simulink library "baro_block_visual"  (R2025b)
settings: Solver=VariableStepAuto  StartTime=0.0  StopTime=10.0  RelTol=1e-3
values from neighbouring files (symbols this model uses):
  Baro = evalin('base', 'Baro')    [casper_baro_step.m]    (also in test_baro_model.m)
  Sim = evalin('base', 'Sim')    [casper_baro_step.m]    (also in test_baro_model.m)
settings Model: Creator=Ashwin  LastModifiedBy=Ashwin

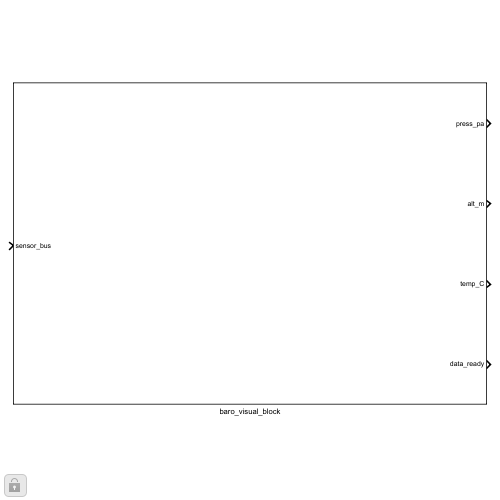
[thumbnail: Simulink's stored preview of the top-level diagram]
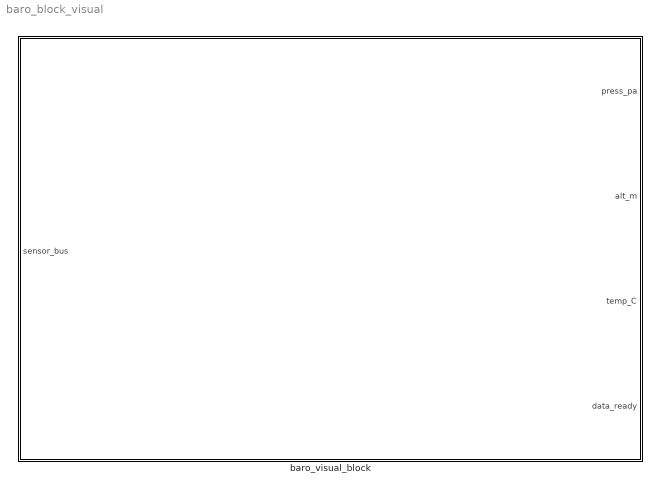
== system baro_block_visual ==
  baro_visual_block : Subsystem

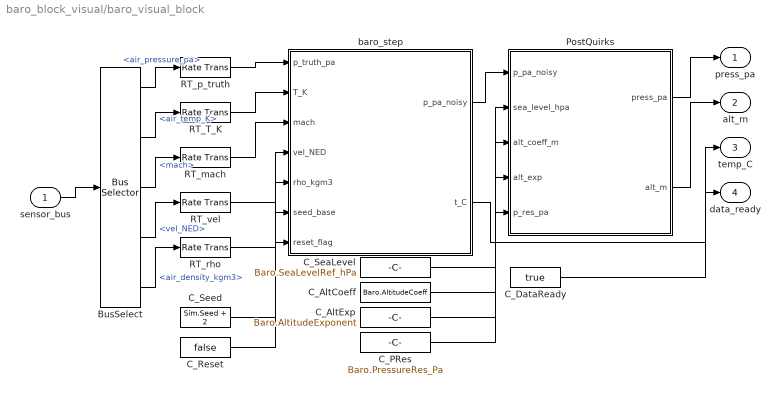
== system baro_block_visual/baro_visual_block ==
  sensor_bus : Inport  OutDataTypeStr=Bus: SensorInputBus
  BusSelect : BusSelector  OutputSignals=air_pressure_pa,air_temp_K,mach,vel_NED,air_density_kgm3
  C_AltCoeff : Constant  Value=Baro.AltitudeCoeff  SampleTime=1/Baro.Rate_Hz
  C_AltExp : Constant  Value=Baro.AltitudeExponent  SampleTime=1/Baro.Rate_Hz
  C_DataReady : Constant  Value=true  OutDataTypeStr=boolean  SampleTime=1/Baro.Rate_Hz
  C_PRes : Constant  Value=Baro.PressureRes_Pa  SampleTime=1/Baro.Rate_Hz
  C_Reset : Constant  Value=false  OutDataTypeStr=boolean  SampleTime=1/Baro.Rate_Hz
  C_SeaLevel : Constant  Value=Baro.SeaLevelRef_hPa  SampleTime=1/Baro.Rate_Hz
  C_Seed : Constant  Value=Sim.Seed + 2  SampleTime=1/Baro.Rate_Hz
  PostQuirks : MATLAB Function  TreatAsAtomicUnit=on
  RT_T_K : RateTransition  OutPortSampleTime=1/Baro.Rate_Hz
  RT_mach : RateTransition  OutPortSampleTime=1/Baro.Rate_Hz
  RT_p_truth : RateTransition  OutPortSampleTime=1/Baro.Rate_Hz
  RT_rho : RateTransition  OutPortSampleTime=1/Baro.Rate_Hz
  RT_vel : RateTransition  OutPortSampleTime=1/Baro.Rate_Hz
  baro_step : MATLAB Function  TreatAsAtomicUnit=on
  press_pa : Outport
  alt_m : Outport  Port=2
  temp_C : Outport  Port=3
  data_ready : Outport  Port=4
  wires:
  sensor_bus/1 -> BusSelect/1
  BusSelect/1 -> RT_p_truth/1  "<air_pressure_pa>"
  BusSelect/2 -> RT_T_K/1  "<air_temp_K>"
  BusSelect/3 -> RT_mach/1  "<mach>"
  BusSelect/4 -> RT_vel/1  "<vel_NED>"
  BusSelect/5 -> RT_rho/1  "<air_density_kgm3>"
  RT_p_truth/1 -> baro_step/1(p_truth_pa)
  RT_T_K/1 -> baro_step/2(T_K)
  RT_mach/1 -> baro_step/3(mach)
  RT_vel/1 -> baro_step/4(vel_NED)
  RT_rho/1 -> baro_step/5(rho_kgm3)
  C_Seed/1 -> baro_step/6(seed_base)
  C_Reset/1 -> baro_step/7(reset_flag)
  baro_step/1(p_pa_noisy) -> PostQuirks/1(p_pa_noisy)
  C_SeaLevel/1 -> PostQuirks/2(sea_level_hpa)
  C_AltCoeff/1 -> PostQuirks/3(alt_coeff_m)
  C_AltExp/1 -> PostQuirks/4(alt_exp)
  C_PRes/1 -> PostQuirks/5(p_res_pa)
  PostQuirks/1(press_pa) -> press_pa/1
  PostQuirks/2(alt_m) -> alt_m/1
  baro_step/2(t_C) -> temp_C/1
  C_DataReady/1 -> data_ready/1

== matlab function baro_block_visual/baro_visual_block/PostQuirks ==
  data: p_pa_noisy input; press_pa output; sea_level_hpa input; alt_coeff_m input; alt_exp input; p_res_pa input; alt_m output
function [press_pa, alt_m] = fcn(p_pa_noisy, sea_level_hpa, alt_coeff_m, alt_exp, p_res_pa)
%#codegen
[press_pa, alt_m] = casper_baro_quirks(p_pa_noisy, sea_level_hpa, alt_coeff_m, alt_exp, p_res_pa);
end

== matlab function baro_block_visual/baro_visual_block/baro_step ==
  data: p_truth_pa input; p_pa_noisy output; T_K input; mach input; vel_NED input; rho_kgm3 input; seed_base input; reset_flag input; t_C output
function [p_pa_noisy, t_C] = fcn(p_truth_pa, T_K, mach, vel_NED, rho_kgm3, seed_base, reset_flag)
coder.extrinsic('casper_baro_step');
p_pa_noisy = double(0);
t_C        = double(0);
[p_pa_noisy, t_C, ~] = casper_baro_step(p_truth_pa, T_K, mach, vel_NED(:), rho_kgm3, double(seed_base), logical(reset_flag));
end
